simulink model "digital_PLL_r2012b"  (Simulink 8.1)
settings: Solver=ode23t  StartTime=0.0  StopTime=8  MaxStep=1e-4  RelTol=1e-4
values from neighbouring files (symbols this model uses):
  K = 0.5    [parametrosPLLMULT.m]
  kc = 712.57    [parametrosPLLMULT.m]
  tauc = 1/wc    (= 0.00266635857081)    [parametrosPLLMULT.m]
  tauz = 1/wz    (= 0.0266635857081)    [parametrosPLLMULT.m]
undefined symbols (not defined in the file or in its folder): SM_of_DigPLLfun
settings Model: Creator=Wassinger  LastModifiedBy=usuario
settings DebuggingCC: StrictBusMsg=Warning

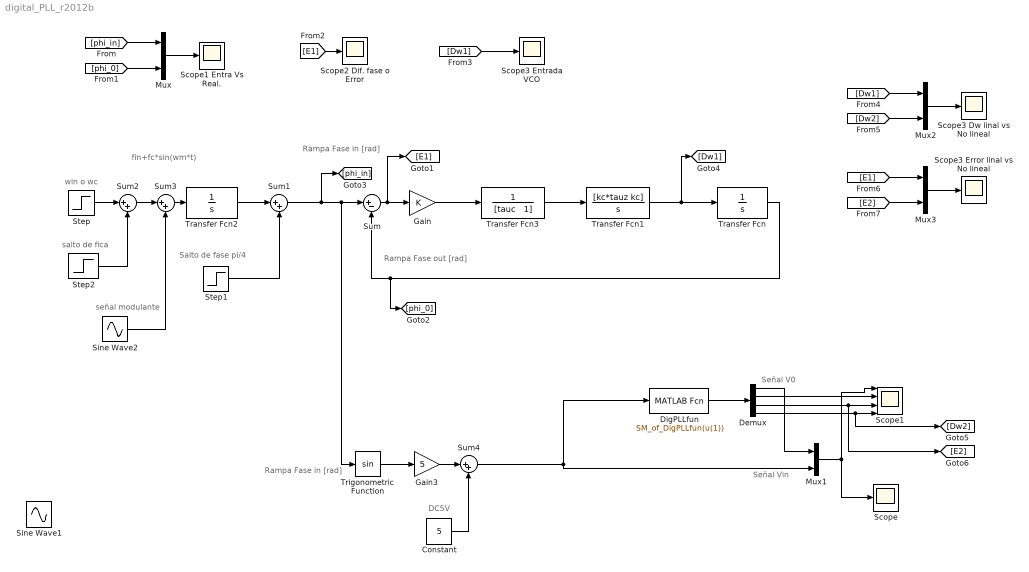
== system digital_PLL_r2012b ==
  note: Señal Vin
  note: Señal V0
  note: Rampa
      | Fase in [rad]
  note: Salto de fase pi/4
  note: fin+fc*sin(wm*t)
  note: señal modulante
  note: win o wc
  note: salto de fica
  note: DC5V
  note: Rampa
      | Fase out [rad]
  note: Rampa
      | Fase in [rad]
  Constant : Constant  Value=5
  Demux : Demux
  DigPLLfun : MATLABFcn  MATLABFcn=SM_of_DigPLLfun(u(1))  OutputDimensions=4  SampleTime=1e-3
  Gain : Gain  Gain=K
  Gain3 : Gain  Gain=5
  Mux{,1..3} (4 alike) : Mux  Inputs=2
  Scope : Scope
      settings: SaveName=ScopeData3
  Scope1 : Scope  NumInputPorts=4
      settings: YMin=-5~-5~-5~-5  YMax=5~5~5~5
  Scope1 Entra Vs Real. : Scope
      settings: AttributesFormatString=%<AxesTitles>  YMin=500  YMax=1550  SaveName=ScopeData4
  Scope2 Dif. fase o Error : Scope
      settings: AttributesFormatString=%<AxesTitles>
  Scope3 Dw linal vs No lineal : Scope
      settings: AttributesFormatString=%<AxesTitles>  SaveName=ScopeData5
  Scope3 Entrada VCO : Scope
      settings: AttributesFormatString=%<AxesTitles>  SaveName=ScopeData2
  Scope3 Error linal vs No lineal : Scope
      settings: AttributesFormatString=%<AxesTitles>  SaveName=ScopeData6
  Sine Wave1 : Sin  Amplitude=5  Bias=5  Frequency=50*2*pi  SampleTime=0
  Sine Wave2 : Sin  Amplitude=0*2*pi*2.5  Frequency=2*pi*7  SampleTime=0
  Step : Step  Time=0  After=2*pi*50  SampleTime=0
  Step1 : Step  Time=4  After=0*pi/4  SampleTime=0
  Step2 : Step  Time=4  Before=0*2*pi*47.5  After=0*2*pi*52.5  SampleTime=0
  Sum : Sum  Inputs=|+-
  Sum{1..4} (4 alike) : Sum  Inputs=|++
  Transfer Fcn : TransferFcn  Numerator=1  Denominator=[1 0]
  Transfer Fcn1 : TransferFcn  Numerator=[kc*tauz kc]  Denominator=[1 0]
  Transfer Fcn2 : TransferFcn  Denominator=[1 0]
  Transfer Fcn3 : TransferFcn  Denominator="[tauc   1]"
  Trigonometric Function : Trigonometry
  wires:
  DigPLLfun/1 -> Demux/1
  Mux1/1 -> Scope/1, Scope1/1
  Demux/1 -> Mux1/1
  Demux/2 -> Scope1/2
  Demux/3 -> [E2], Scope1/3
  Demux/4 -> [Dw2], Scope1/4
  Transfer Fcn2/1 -> Sum1/1
  Step1/1 -> Sum1/2
  Step/1 -> Sum2/1
  Step2/1 -> Sum2/2
  Sum2/1 -> Sum3/1
  Sine Wave2/1 -> Sum3/2
  Sum3/1 -> Transfer Fcn2/1
  Sum1/1 -> [phi_in], Trigonometric Function/1, Sum/1
  Trigonometric Function/1 -> Gain3/1
  Gain3/1 -> Sum4/1
  Constant/1 -> Sum4/2
  Sum4/1 -> DigPLLfun/1, Mux1/2
  Transfer Fcn1/1 -> [Dw1], Transfer Fcn/1
  Transfer Fcn/1 -> [phi_0], Sum/2
  Gain/1 -> Transfer Fcn3/1
  Sum/1 -> [E1], Gain/1
  Transfer Fcn3/1 -> Transfer Fcn1/1
  [phi_in] -> Mux/1
  [phi_0] -> Mux/2
  Mux/1 -> Scope1 Entra Vs Real./1
  [E1] -> Scope2 Dif. fase o Error/1
  [Dw1] -> Scope3 Entrada VCO/1
  [Dw2] -> Mux2/2
  Mux2/1 -> Scope3 Dw linal vs No lineal/1
  [E2] -> Mux3/2
  Mux3/1 -> Scope3 Error linal vs No lineal/1
  [Dw1] -> Mux2/1
  [E1] -> Mux3/1
